simulink model "Lab2P2"  (R2021b)
settings: Solver=VariableStepAuto  StartTime=0.0  StopTime=25  RelTol=1e-7
libraries: simulink x1
settings Model: Creator=Ahmad  LastModifiedBy=Ahmad

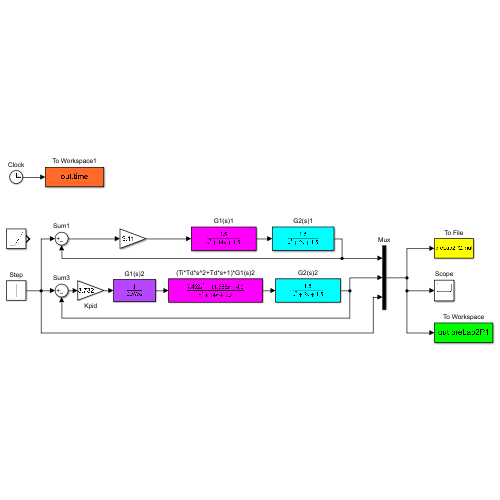
[thumbnail: Simulink's stored preview of the top-level diagram]
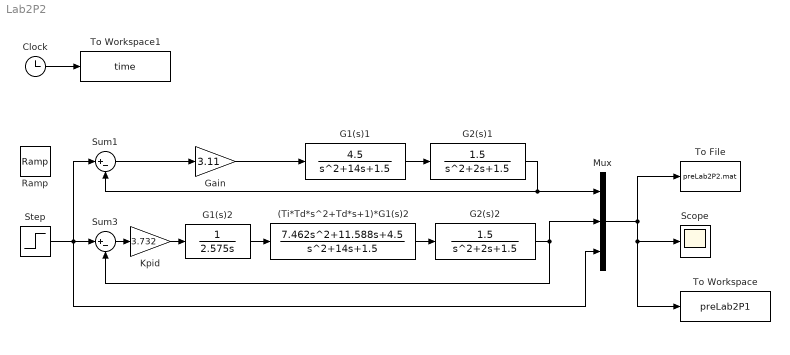
== system Lab2P2 ==
  (Ti*Td*s^2+Td*s+1)*G1(s)2 : TransferFcn  Numerator=[7.462 11.588 4.5]  Denominator=[1 14 1.5]
  Clock : Clock
  G1(s)1 : TransferFcn  Numerator=[4.5]  Denominator=[1 14 1.5]
  G1(s)2 : TransferFcn  Denominator=[2.575 0]
  G2(s)1 : TransferFcn  Numerator=[1.5]  Denominator=[1 2 1.5]
  G2(s)2 : TransferFcn  Numerator=[1.5]  Denominator=[1 2 1.5]
  Gain : Gain  Gain=3.11
  Kpid : Gain  Gain=3.732
  Mux : Mux  Inputs=3
  Ramp : simulink/Sources/Ramp  slope=1  start=0  InitialOutput=0
  Scope : Scope
  Step : Step  Time=0  SampleTime=0
  Sum1 : Sum  Inputs=|+-
  Sum3 : Sum  Inputs=|+-
  To File : ToFile  Filename=preLab2P2.mat  MatrixName=out
  To Workspace : ToWorkspace  VariableName=preLab2P1  SampleTime=-1
  To Workspace1 : ToWorkspace  VariableName=time  SampleTime=-1
  wires:
  Clock/1 -> To Workspace1/1
  Gain/1 -> G1(s)1/1
  Sum1/1 -> Gain/1
  G1(s)1/1 -> G2(s)1/1
  (Ti*Td*s^2+Td*s+1)*G1(s)2/1 -> G2(s)2/1
  Mux/1 -> To Workspace/1, Scope/1, To File/1
  G2(s)1/1 -> Sum1/2, Mux/1
  G2(s)2/1 -> Mux/2, Sum3/2
  Step/1 -> Sum3/1, Mux/3, Sum1/1
  Sum3/1 -> Kpid/1
  G1(s)2/1 -> (Ti*Td*s^2+Td*s+1)*G1(s)2/1
  Kpid/1 -> G1(s)2/1
